simulink model "pv_to_resis_load"  (R2022a)
settings: Solver=VariableStepAuto  StartTime=0.0  StopTime=1  RelTol=1e-3
libraries: spsSeriesRLCBranchLib x15, spsMosfetLib x6, eeRmsMeasurement x5, simulink x3, spsCurrentMeasurementLib x2, spsGroundLib x2, spsMeanLib x2, spsVoltageMeasurementLib x2, spsDiodeLib x1, spsIGBTDiodeLib x1, slpidlib x1, spsPVArrayLib x1
settings Model: Creator=eee  LastModifiedBy=eee

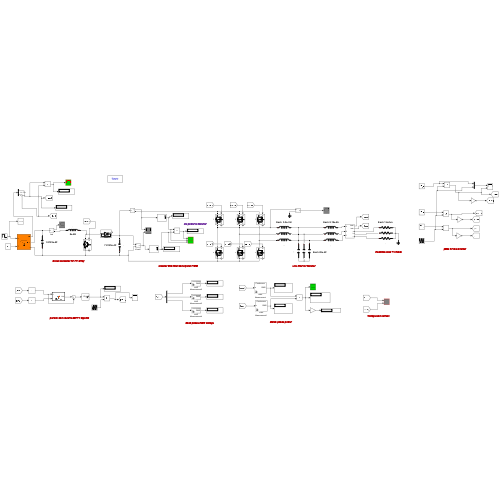
[thumbnail: Simulink's stored preview of the top-level diagram]
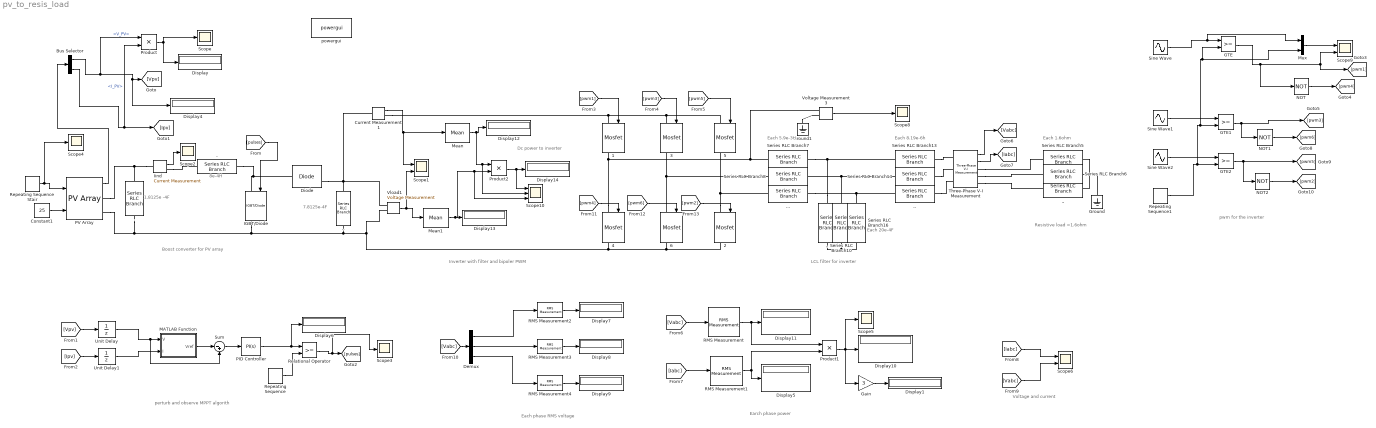
== system pv_to_resis_load ==
  note: Boost converter for PV array
  note: Inverter with filter and bipoler PWM
  note: LCL filter for inverter
  note: Resistive load =1.6ohm
  note: Voltage and current
  note: Earch phase power
  note: Each phase RMS voltage
  note: perturb and observe MPPT algorith
  note: 1.8125e -4F
  note: 8e-4H
  note: 7.8125e-4F
  note: Dc power to inverter
  note: Each 5.9e-3H
  note: Each 20e-4F
  note: Each 8.19e-6h
  note: Each 1.6ohm
  note: pwm for the inverter
  , : spsSeriesRLCBranchLib/Series RLC Branch  LConnTagsString=__new0  RConnTagsString=__new0  BranchType=L  Resistance=1e-3  Inductance=8e-4  SetiL0=off  InitialCurrent=0  Capacitance=1000e-6  Setx0=off  InitialVoltage=0  Measurements=None
  ,, : spsSeriesRLCBranchLib/Series RLC Branch  LConnTagsString=__new0  RConnTagsString=__new0  BranchType=C  Resistance=2.941  Inductance=1e-3  SetiL0=off  InitialCurrent=0  Capacitance=20e-4  Setx0=off  InitialVoltage=0  Measurements=None
  ,. : spsSeriesRLCBranchLib/Series RLC Branch  LConnTagsString=__new0  RConnTagsString=__new0  BranchType=L  Resistance=2.941  Inductance=8.19e-6  SetiL0=off  InitialCurrent=0  Capacitance=2  Setx0=off  InitialVoltage=0  Measurements=None
  . : spsSeriesRLCBranchLib/Series RLC Branch  LConnTagsString=__new0  RConnTagsString=__new0  BranchType=C  Resistance=1e-3  Inductance=1.45e-3  SetiL0=off  InitialCurrent=0  Capacitance=1.8125e-4  Setx0=off  InitialVoltage=0  Measurements=None
  ., : spsSeriesRLCBranchLib/Series RLC Branch  LConnTagsString=__new0  RConnTagsString=__new0  BranchType=R  Resistance=1.6  Inductance=2.828e-4  SetiL0=off  InitialCurrent=0  Capacitance=2  Setx0=off  InitialVoltage=0  Measurements=None
  .. : spsSeriesRLCBranchLib/Series RLC Branch  LConnTagsString=__new0  RConnTagsString=__new0  BranchType=C  Resistance=1e-3  Inductance=1.45e-3  SetiL0=off  InitialCurrent=0  Capacitance=7.8125e-4  Setx0=off  InitialVoltage=0  Measurements=None
  ... : spsSeriesRLCBranchLib/Series RLC Branch  LConnTagsString=__new0  RConnTagsString=__new0  BranchType=L  Resistance=2.941  Inductance=5.9e-3  SetiL0=off  InitialCurrent=0  Capacitance=2  Setx0=off  InitialVoltage=0  Measurements=None
  {1..6} (6 alike) : spsMosfetLib/Mosfet  Ron=0.1  Lon=0  Rd=0.01  Vfd=0  IC=0  Rs=1e5  Cs=inf  Measurements=on
  Bus Selector : BusSelector  OutputSignals=V_PV,I_PV
  Constant1 : Constant  Value=25
  Current Measurement1 : spsCurrentMeasurementLib/Current Measurement  PhasorSimulation=off  OutputType=Complex  PSBequivalent=0
  Demux : Demux  Outputs=3
  Diode : spsDiodeLib/Diode  Ron=0.001  Lon=0  Vf=0.8  IC=0  UseSnubber=0  Rs=500  Cs=250e-9  Measurements=on
  Display{,1,4..14} (13 alike) : Display
  GTE : RelationalOperator  OutDataTypeStr=boolean  RndMeth=Simplest  InputSameDT=off
  GTE1 : RelationalOperator  OutDataTypeStr=boolean  RndMeth=Simplest  InputSameDT=off
  GTE2 : RelationalOperator  OutDataTypeStr=boolean  RndMeth=Simplest  InputSameDT=off
  Gain : Gain  Gain=3
  Ground : spsGroundLib/Ground  LConnTagsString=a
  Ground1 : spsGroundLib/Ground  LConnTagsString=a
  IGBT/Diode : spsIGBTDiodeLib/IGBT//Diode  Ron=1e-3  Rs=1e5  Cs=inf  Measurements=on
  Iind : spsCurrentMeasurementLib/Current Measurement  PhasorSimulation=off  OutputType=Complex  PSBequivalent=0
  MATLAB Function : MATLAB Function  TreatAsAtomicUnit=on
  Mean : spsMeanLib/Mean  Freq=50  Vinit=0  Ts=0
  Mean1 : spsMeanLib/Mean  Freq=50  Vinit=0  Ts=0
  Mux : Mux  Inputs=2
  NOT : Logic  Operator=NOT  IconShape=distinctive  AllPortsSameDT=off  OutDataTypeStr=boolean
  NOT1 : Logic  Operator=NOT  IconShape=distinctive  AllPortsSameDT=off  OutDataTypeStr=boolean
  NOT2 : Logic  Operator=NOT  IconShape=distinctive  AllPortsSameDT=off  OutDataTypeStr=boolean
  PID Controller : slpidlib/PID Controller  Controller=PI  Form=Parallel  TimeDomain=Continuous-time  UseExternalTs=off  SampleTime=-1  IntegratorMethod=Forward Euler  FilterMethod=Forward Euler  ControllerParametersSource=internal  P=0.001  I=0.01  UseKiTs=off  D=0  N=100  UseFilter=on  TunerSelectOption=Transfer Function Based (PID Tuner App)  InitialConditionSource=internal  InitialConditionForIntegrator=0  InitialConditionForFilter=0  DifferentiatorICPrevScaledInput=0  ExternalReset=none  TrackingMode=off  Kt=1  LimitOutput=on  SatLimitsSource=internal  UpperSaturationLimit=0.95  LowerSaturationLimit=0  LinearizeAsGain=on  AntiWindupMode=none  Kb=1  POutMin=[]  POutMax=[]  IOutMin=[]  IOutMax=[]  DOutMin=[]  DOutMax=[]  NOutMin=[]  NOutMax=[]  SumOutMin=[]  SumOutMax=[]  SaturationOutMin=[]  SaturationOutMax=[]  PParamMin=[]  PParamMax=[]  IParamMin=[]  IParamMax=[]  DParamMin=[]  DParamMax=[]  NParamMin=[]  NParamMax=[]  KbParamMin=[]  KbParamMax=[]  KtParamMin=[]  KtParamMax=[]  KbOutMin=[]  KbOutMax=[]  KtOutMin=[]  KtOutMax=[]  IntegratorOutMin=[]  IntegratorOutMax=[]  FilterOutMin=[]  FilterOutMax=[]  SumI1OutMin=[]  SumI1OutMax=[]  SumI2OutMin=[]  SumI2OutMax=[]  SumI3OutMin=[]  SumI3OutMax=[]  SumI4OutMin=[]  SumI4OutMax=[]  SumDOutMin=[]  SumDOutMax=[]  DifferentiatorOutMin=[]  DifferentiatorOutMax=[]  FilterDiffOutCoefMin=[]  FilterDiffOutCoefMax=[]  ReciprocalOutMin=[]  ReciprocalOutMax=[]  SumDenOutMin=[]  SumDenOutMax=[]  SumNumOutMin=[]  SumNumOutMax=[]  DivideOutMin=[]  DivideOutMax=[]  UdiffTsProdOutMin=[]  UdiffTsProdOutMax=[]  NTsProdOutMin=[]  NTsProdOutMax=[]  UintegralTsProdOutMin=[]  UintegralTsProdOutMax=[]  UngainTsProdOutMin=[]  UngainTsProdOutMax=[]  IntegratorContinuousStateAttributes=''  IntegratorStateMustResolveToSignalObject=off  IntegratorRTWStateStorageClass=Auto  FilterContinuousStateAttributes=''  FilterStateMustResolveToSignalObject=off  FilterRTWStateStorageClass=Auto  ParallelPVariant=InternalParameters  IdealPVariant=Disabled  IVariant=InternalParameters  DVariant=Disabled  IntegratorVariant=Continuous  SatVariant=Enabled  AWVariant=Passthrough  PCopyVariant=Disabled  TRVariant=Disabled  FdbkBlocksVariant=Forward  IdealPFdbkVariant=Disabled  SatFdbkVariant=Disabled  DerivativeFilterVariant=Disabled  NVariant=Disabled  NCopyVariant=Disabled_SignalSpec  FilterICVariant=Disabled  IntegratorICVariant=InternalICs  ExternalResetVariant=Disabled  TRSumVariant=Passthrough  SumFdbkVariant=Disabled  SumVariant=Sum_PI  TsampFilterVariant=InternalTs  TsampNgainVariant=Passthrough  TsampIntegralVariant=Passthrough  ExternalSaturationOutDataTypeStr=Inherit: Same as second input  aMode=0
  PV Array : spsPVArrayLib/PV Array  Npar=34  Nser=14  PlotType=array @ 1000 W/m2 & specified temperatures  S_vec="[ 1000  500  100 ]"  Temp_C_vec="[ 45 25  ]"  ModuleName=SOLTON Power SPI-215P  PlotWhenSelected=off  Pm=214.858  Ncell=60  Voc=36.12  Isc=7.74  Vm=29.8  Im=7.21  beta_Voc_pc=-0.33  alpha_Isc_pc=0.05  beta_Voc=-0.1192  alpha_Isc=0.00387  IL=7.7519  I0=8.6507e-11  nI=0.9301  Rsh=178.006  Rs=0.27329  RobustModel=off  RobustCellTemperature=313.3991  BAL=on  Tc=1e-6  Tfilter=5e-5
  Product : Product
  Product1 : Product
  Product2 : Product
  RMS Measurement{,1..4} (5 alike) : eeRmsMeasurement/RMS Measurement  LabelModeActiveChoice=Total  F=50  SpecifyHarmonics=off  K=[0 1 2]  Ts=0
      settings: SourceProductBaseCode=PS
  Relational Operator : RelationalOperator  OutDataTypeStr=boolean  RndMeth=Simplest  InputSameDT=off
  Repeating Sequence : simulink/Sources/Repeating Sequence  rep_seq_t=[0 0.0001]  rep_seq_y=[0 1]
  Repeating Sequence Stair : simulink/Sources/Repeating Sequence Stair  OutValues=[1000 500].'  tsamp=3  OutMin=[]  OutMax=[]  OutDataTypeStr=double  OutputDataTypeScalingMode=double  OutDataType=fixdt(0,8)  ConRadixGroup=Best Precision: Vector-wise  OutScaling=2^-12
  Repeating Sequence1 : simulink/Sources/Repeating Sequence  rep_seq_t=[0 1 2 3 4]*[1/10000]  rep_seq_y=[0 1 0 -1 0]
  Scope{,2..5,8} (6 alike) : Scope
  Scope1 : Scope  NumInputPorts=2
  Scope10 : Scope  NumInputPorts=3
  Scope6 : Scope  NumInputPorts=2
  Scope9 : Scope  NumInputPorts=2
  Series RLC Branch10 : spsSeriesRLCBranchLib/Series RLC Branch  LConnTagsString=__new0  RConnTagsString=__new0  BranchType=C  Resistance=2.941  Inductance=1e-3  SetiL0=off  InitialCurrent=0  Capacitance=20e-4  Setx0=off  InitialVoltage=0  Measurements=None
  Series RLC Branch13 : spsSeriesRLCBranchLib/Series RLC Branch  LConnTagsString=__new0  RConnTagsString=__new0  BranchType=L  Resistance=2.941  Inductance=8.19e-6  SetiL0=off  InitialCurrent=0  Capacitance=2  Setx0=off  InitialVoltage=0  Measurements=None
  Series RLC Branch14 : spsSeriesRLCBranchLib/Series RLC Branch  LConnTagsString=__new0  RConnTagsString=__new0  BranchType=L  Resistance=2.941  Inductance=8.19e-6  SetiL0=off  InitialCurrent=0  Capacitance=2  Setx0=off  InitialVoltage=0  Measurements=None
  Series RLC Branch16 : spsSeriesRLCBranchLib/Series RLC Branch  LConnTagsString=__new0  RConnTagsString=__new0  BranchType=C  Resistance=2.941  Inductance=1e-3  SetiL0=off  InitialCurrent=0  Capacitance=20e-4  Setx0=off  InitialVoltage=0  Measurements=None
  Series RLC Branch5 : spsSeriesRLCBranchLib/Series RLC Branch  LConnTagsString=__new0  RConnTagsString=__new0  BranchType=R  Resistance=1.6  Inductance=2.828e-4  SetiL0=off  InitialCurrent=0  Capacitance=2  Setx0=off  InitialVoltage=0  Measurements=None
  Series RLC Branch6 : spsSeriesRLCBranchLib/Series RLC Branch  LConnTagsString=__new0  RConnTagsString=__new0  BranchType=R  Resistance=1.6  Inductance=2.828e-4  SetiL0=off  InitialCurrent=0  Capacitance=2  Setx0=off  InitialVoltage=0  Measurements=None
  Series RLC Branch7 : spsSeriesRLCBranchLib/Series RLC Branch  LConnTagsString=__new0  RConnTagsString=__new0  BranchType=L  Resistance=2.941  Inductance=5.9e-3  SetiL0=off  InitialCurrent=0  Capacitance=2  Setx0=off  InitialVoltage=0  Measurements=None
  Series RLC Branch8 : spsSeriesRLCBranchLib/Series RLC Branch  LConnTagsString=__new0  RConnTagsString=__new0  BranchType=L  Resistance=2.941  Inductance=5.9e-3  SetiL0=off  InitialCurrent=0  Capacitance=2  Setx0=off  InitialVoltage=0  Measurements=None
  Sine Wave : Sin  Frequency=2*pi*50  SampleTime=0
  Sine Wave1 : Sin  Frequency=2*pi*50  Phase=pi/180*120  SampleTime=0
  Sine Wave2 : Sin  Frequency=2*pi*50  Phase=pi/180*240  SampleTime=0
  Sum : Sum  Inputs=|-+
  Three-Phase V-I Measurement : spsThreePhaseVIMeasurementLib/Three-Phase V-I Measurement  VoltageMeasurement=phase-to-ground  SetLabelV=off  LabelV=Vabc  Vpu=off  VpuLL=off  CurrentMeasurement=yes  SetLabelI=off  LabelI=Iabc  Ipu=off  Pbase=100e6  Vbase=500e3  OutputType=Complex  PhasorSimulation=off  PSBequivalent=0
  Unit Delay : UnitDelay  SampleTime=1e-4  HasFrameUpgradeWarning=on
  Unit Delay1 : UnitDelay  SampleTime=1e-4  HasFrameUpgradeWarning=on
  Vload1 : spsVoltageMeasurementLib/Voltage Measurement  PhasorSimulation=off  OutputType=Complex  PSBequivalent=0
  Voltage Measurement3 : spsVoltageMeasurementLib/Voltage Measurement  PhasorSimulation=off  OutputType=Complex  PSBequivalent=0
  powergui : spspowerguiLib/powergui  Priority=1  SimulationMode=Discrete  SampleTime=1e-6  frequency=60  Iterations=50  frequencyindice=0  Pbase=100e6  ErrMax=1e-4  UnitsV=kV  UnitsW=MW  buscounter=0  FunctionMessages=off  echomessages=off  EnableUseOfTLC=off  CurrentSourceSwitches=off  DisableSnubberDevices=off  DisableRonSwitches=off  DisableVfSwitches=off  DisplayEquations=off  AutomaticDiscreteSolvers=off  SolverType=Tustin/Backward Euler (TBE)  Interpol=off  ExternalGateDelay=off  methode=off  Ts=100  x0status=blocks  SPID=on  SwTol=0  HookPort=off  NonlinearTolerance=1e-4  nMaxIteration=100  ContinueOnMaxIteration=off  RestoreLinks=warning  ResistiveCurrentMeasurement=off  Frange=[0:2:500]  Ylog=off  Xlog=on  ShowGrid=off  save=off  variable=ZData  structure=0  ZoomFFT=off  StartTime=0.0  cycles=1  DisplayStyle=1  fundamental=60  FreqAxis=off  MaxFrequency=1000  frequencyindicesteady=1  RmsSteady=1  display=off
  wires:
  PV Array/1 -> Bus Selector/1
  Repeating Sequence Stair/1 -> Scope4/1, PV Array/1
  MATLAB Function/1(Vref) -> Sum/1
  [pulses] -> IGBT/Diode/1
  Relational Operator/1 -> Scope3/1, [pulses]
  Repeating Sequence/1 -> Relational Operator/2
  Sum/1 -> PID Controller/1
  PID Controller/1 -> Display6/1, Relational Operator/1
  [Ipv] -> Unit Delay1/1
  Bus Selector/2 -> Product/2, [Ipv]  "<I_PV>"
  Bus Selector/1 -> Display4/1, [Vpv], Product/1  "<V_PV>"
  Unit Delay1/1 -> MATLAB Function/2(I)
  Constant1/1 -> PV Array/2
  [Vpv] -> Unit Delay/1
  Product/1 -> Display/1, Scope/1
  Iind/1 -> Scope2/1
  Unit Delay/1 -> Sum/2, MATLAB Function/1(V)
  Demux/2 -> RMS Measurement3/1
  RMS Measurement4/1 -> Display9/1
  Demux/1 -> RMS Measurement2/1
  RMS Measurement3/1 -> Display8/1
  Demux/3 -> RMS Measurement4/1
  [Vabc] -> Demux/1
  Product1/1 -> Gain/1, Display10/1, Scope5/1
  [Vabc] -> RMS Measurement/1
  RMS Measurement/1 -> Product1/1, Display11/1
  [Iabc] -> RMS Measurement1/1
  RMS Measurement1/1 -> Display5/1, Product1/2
  [Iabc] -> Scope6/1
  [Vabc] -> Scope6/2
  Three-Phase V-I Measurement/2 -> [Iabc]
  Three-Phase V-I Measurement/1 -> [Vabc]
  [pwm5] -> 5/1
  Current Measurement1/1 -> Scope1/1, Mean/1
  Voltage Measurement3/1 -> Scope8/1
  [pwm6] -> 6/1
  [pwm3] -> 3/1
  [pwm1] -> 1/1
  [pwm4] -> 4/1
  Mean/1 -> Scope10/2, Product2/1, Display12/1
  [pwm2] -> 2/1
  NOT1/1 -> [pwm6]
  NOT/1 -> [pwm4]
  NOT2/1 -> [pwm2]
  Repeating Sequence1/1 -> Mux/2, GTE/2, GTE1/2, GTE2/2
  GTE2/1 -> NOT2/1, [pwm5]
  Sine Wave/1 -> Mux/1, GTE/1
  GTE/1 -> NOT/1, [pwm1], Scope9/2
  Mux/1 -> Scope9/1
  GTE1/1 -> NOT1/1, [pwm3]
  Sine Wave1/1 -> GTE1/1
  Sine Wave2/1 -> GTE2/1
  Vload1/1 -> Scope1/2, Mean1/1
  Mean1/1 -> Scope10/3, Product2/2, Display13/1
  Product2/1 -> Scope10/1, Display14/1
  RMS Measurement2/1 -> Display7/1
  Gain/1 -> Display1/1
  connections:
  ,/LConn1 -- IGBT/Diode/LConn1 -- Diode/LConn1
  Iind/LConn1 -- ./RConn1 -- PV Array/RConn1
  Diode/RConn1 -- ../RConn1 -- Vload1/LConn1 -- Current Measurement1/LConn1
  Iind/RConn1 -- ,/RConn1
  .,/RConn1 -- Ground/LConn1 -- Series RLC Branch5/RConn1 -- Series RLC Branch6/RConn1
  Series RLC Branch16/LConn1 -- ,./LConn1 -- .../RConn1
  4/LConn1 -- 1/RConn1 -- Voltage Measurement3/LConn1 -- Series RLC Branch7/LConn1
  PV Array/RConn2 -- IGBT/Diode/RConn1 -- Vload1/LConn2 -- 2/RConn1 -- 6/RConn1 -- 4/RConn1 -- ../LConn1 -- ./LConn1
  Series RLC Branch8/LConn1 -- 3/RConn1 -- 6/LConn1
  Series RLC Branch10/RConn1 -- Series RLC Branch16/RConn1 -- ,,/RConn1
  ,,/LConn1 -- Series RLC Branch7/RConn1 -- Series RLC Branch13/LConn1
  2/LConn1 -- 5/RConn1 -- .../LConn1
  Series RLC Branch8/RConn1 -- Series RLC Branch14/LConn1 -- Series RLC Branch10/LConn1
  1/LConn1 -- 3/LConn1 -- 5/LConn1 -- Current Measurement1/RConn1
  Three-Phase V-I Measurement/RConn1 -- Series RLC Branch5/LConn1
  Three-Phase V-I Measurement/RConn2 -- Series RLC Branch6/LConn1
  Three-Phase V-I Measurement/RConn3 -- .,/LConn1
  ,./RConn1 -- Three-Phase V-I Measurement/LConn3
  Series RLC Branch14/RConn1 -- Three-Phase V-I Measurement/LConn2
  Series RLC Branch13/RConn1 -- Three-Phase V-I Measurement/LConn1
  Voltage Measurement3/LConn2 -- Ground1/LConn1

== matlab function pv_to_resis_load/MATLAB Function ==
  data: V input; Vref output; I input
% Perturb AND observe  MPPT
function Vref = RefGen(V,I)
Vrefmax=450;
Vrefmin=0;
Vrefinit=300;
deltaVref=1;
persistent Vold Pold Vrefold;
dataType = 'double'
if isempty(Vold)
    Vold =0;
    Pold=0;
    Vrefold=Vrefinit;
end
P=V*I;
dV=V-Vold;
dP=P-Pold;
if dP~=0
    if dP<0
        if dV<0
            Vref=Vrefold+deltaVref;
        else
        Vref=Vrefold-deltaVref;
        end
else
    if dV<0
        Vref=Vrefold-deltaVref;
    else
        Vref=Vrefold+deltaVref;
    end
    end
else
    Vref = Vrefold;
end
if Vref>=Vrefmax | Vref<=Vrefmin
    Vref=Vrefold;
end
Vrefold=Vref;
Vold=V;
Pold=P;
